simulink model "c2837xD_lcd_display"  (R2021b)
settings: Solver=FixedStepDiscrete  StartTime=0.0  StopTime=Inf  RelTol=1e-3  EnableMultiTasking=on
InitFcn:
  | c2837xD_Display_Param;
values from neighbouring files (symbols this model uses):
  SCI_counter = SCI_ping_buffer_size/SCI_chunk_size    (= 640)    [c2837xD_Display_Param.m]
  SCI_ping_buffer_size = image_height*lines_in_packet    (= 3840)    [c2837xD_Display_Param.m]
  TI_chunk_size = SCI_chunk_size    (= 6)    [c2837xD_Display_Param.m]
  TI_ping_buffer_size = SCI_ping_buffer_size    (= 3840)    [c2837xD_Display_Param.m]
libraries: c280xlib x63, c2837xDlib x63, simulink x41, c2000lib x1, demo_controls x1, dspswit3 x1, idelinklib_common x1
(part 1 of 4)
CloseFcn:
  | clearvars Image_Array image_height image_width lines_in_packet;
  | clearvars SCI_chunk_size SCI_counter SCI_ping_buffer_size;
  | clearvars SPI_chunk_size TI_chunk_size TI_ping_buffer_size;
  | clearvars ACK_array ACK_watchdog delimiter;
  | clearvars I IB IG Image inc1 inc2 IR IRG IRGB serial_obj CurrentBufferData CurrentBuffercount;
settings Model: ExtModeTrigDuration=8  Creator=The MathWorks, Inc.  LastModifiedBy=The MathWorks, Inc.
settings SolverCC: AlgebraicLoopSolver=TrustRegion
settings DataIOCC: ReturnWorkspaceOutputs=off
settings OptimizationCC: DefaultUnderspecifiedDataType=single  PassReuseOutputArgsAs=Individual arguments  MaxStackSize=512  EfficientTunableParamExpr=on
settings DebuggingCC: InheritedTsInSrcMsg=none  ParameterTunabilityLossMsg=error  SFMachineParentedDataDiag=warning  ArithmeticOperatorsInVariantConditions=warning
settings HardwareCC: ProdBitPerChar=16  ProdBitPerInt=16  ProdBitPerPointer=32  ProdBitPerSizeT=32  ProdBitPerPtrDiffT=32  ProdLargestAtomicInteger=Integer  ProdLargestAtomicFloat=None  ProdWordSize=16  ProdLongLongMode=on  ProdHWDeviceType=Texas Instruments->C2000
settings SFSimCC: SimUseLocalCustomCode=off  MATLABDynamicMemAlloc=off  CustomCodeUndefinedFunction=UseInterfaceOnly
settings RTWCC: Description=Embedded Coder  SystemTargetFile=ert.tlc  HardwareBoard=TI Delfino F28379D LaunchPad  TemplateMakefile=ert_default_tmf  GenerateReport=on  RTWUseLocalCustomCode=off  Toolchain=Texas Instruments Code Composer Studio (C2000)  IncludeHyperlinkInReport=on  LaunchReport=on  GenerateTraceInfo=on  GenerateTraceReport=on  GenerateTraceReportSl=on  GenerateTraceReportSf=on  GenerateTraceReportEml=on
settings CodeAppCC: ForceParamTrailComments=on  IgnoreCustomStorageClasses=off  OperatorAnnotations=on  SimulinkDataObjDesc=on  SFDataObjDesc=on  InsertBlockDesc=on
settings ERTTargetCC: CodeReplacementLibrary=TI C28x  MemSecPackage=tic2000demospkg  MemSecFuncExecute=code_ramfuncs

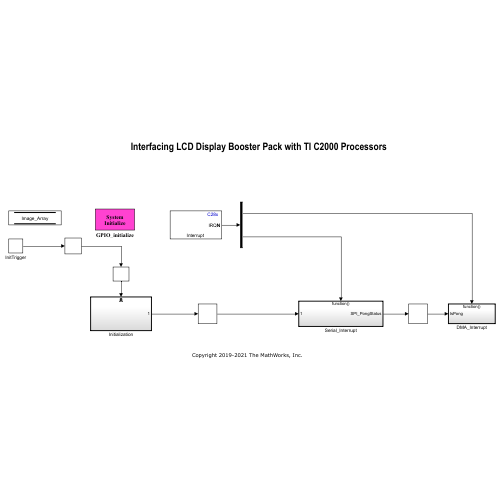
[thumbnail: Simulink's stored preview of the top-level diagram]
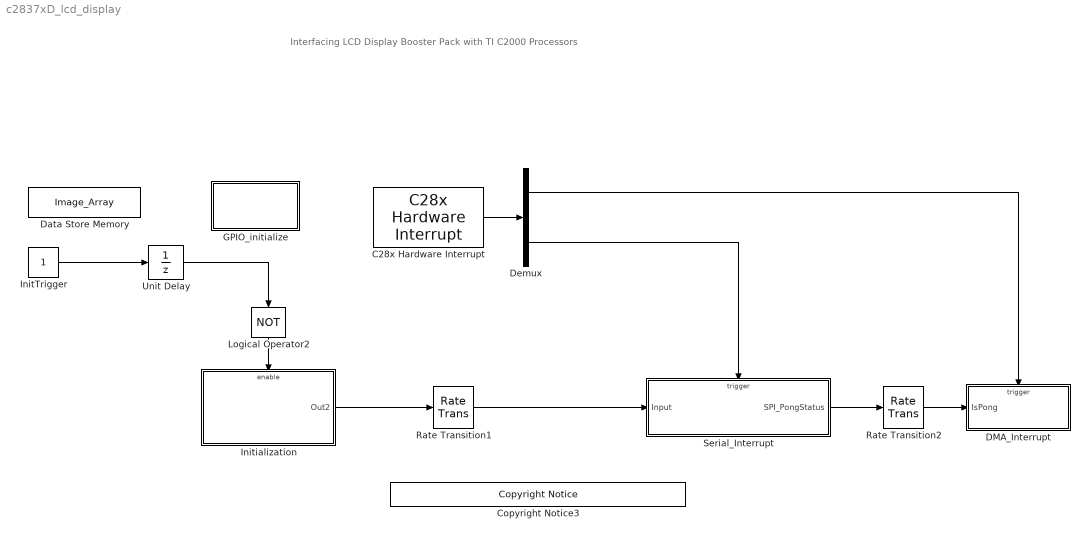
== system c2837xD_lcd_display ==
  note: Interfacing LCD Display Booster Pack with TI C2000 Processors
  C28x Hardware Interrupt : c2000lib/Scheduling/C28x Hardware Interrupt  irqnumbers=[7 9]  pienumbers=[1 1]  irqpriorities=[30 31]  irqpreempts=[1 0]  showinput=off  dspchiptype=C280X
      settings: SourceProductBaseCode=TIC2000
  Copyright Notice3 : demo_controls/Copyright Notice  year=2019  prod=tic2000
      settings: SourceProductBaseCode=ME
  DMA_Interrupt : Subsystem  TreatAsAtomicUnit=on
  Data Store Memory : DataStoreMemory  DataStoreName=Image_Array  ReadBeforeWriteMsg=warning  WriteAfterWriteMsg=warning  WriteAfterReadMsg=warning  InitialValue=[]  ShowAdditionalParam=off  OutDataTypeStr=uint16  Dimensions=SCI_ping_buffer_size*2  StateMustResolveToSignalObject=on
  Demux : Demux  Outputs=2
  GPIO_initialize : Subsystem  mask(System Initialize){ShowInLibBrowser=0}
      mask prompts: ShowInLibBrowser "Simulink:masks:CustCodeMaskParam1_MP"
      settings: CopyFcn=cccopyfcn(gcb)  OpenFcn=ccopenfcn('System Initialize Function')
      mask Help: eval('feval(''rtwprivate'',''rtwhelpview'',''rtw_sys_initialize_block'')');
      mask Display: disp('System\nInitialize');
  InitTrigger : Constant  OutDataTypeStr=uint16  SampleTime=0.1
  Initialization : Subsystem
  Logical Operator2 : Logic  Priority=2  Operator=NOT  AllPortsSameDT=off  OutDataTypeStr=boolean
  Rate Transition1 : RateTransition  Integrity=off
  Rate Transition2 : RateTransition  Integrity=off
  Serial_Interrupt : Subsystem  TreatAsAtomicUnit=on
      settings: RTWSystemCode=Nonreusable function
  Unit Delay : UnitDelay  Priority=1  SampleTime=-1  HasFrameUpgradeWarning=on
  wires:
  Initialization/1(Out2) -> Rate Transition1/1
  Demux/1 -> DMA_Interrupt/Trigger
  Demux/2 -> Serial_Interrupt/Trigger
  Logical Operator2/1 -> Initialization/Enable
  Unit Delay/1 -> Logical Operator2/1
  Rate Transition1/1 -> Serial_Interrupt/1(Input)
  InitTrigger/1 -> Unit Delay/1
  C28x Hardware Interrupt/1 -> Demux/1
  Serial_Interrupt/1(SPI_PongStatus) -> Rate Transition2/1
  Rate Transition2/1 -> DMA_Interrupt/1(IsPong)

== system c2837xD_lcd_display/DMA_Interrupt ==
  IsPong : Inport
  function : TriggerPort  TriggerType=function-call  VariantControl=Variant
  ACKCounter : simulink/Sources/Counter Free-Running  NumBits=16  tsamp=-1
  NOT : Logic  Operator=NOT  IconShape=distinctive  AllPortsSameDT=off  OutDataTypeStr=boolean
  SCI Transmit : c280xlib/SCI Transmit  sciModule=A  dataHead='S'  dataTail='E'  postInterrupt=off  numFifo=1
  Subsystem : Subsystem
  Subsystem1 : Subsystem
  wires:
  ACKCounter/1 -> SCI Transmit/1
  IsPong/1 -> Subsystem1/Enable, NOT/1
  NOT/1 -> Subsystem/Enable

== system c2837xD_lcd_display/GPIO_initialize ==

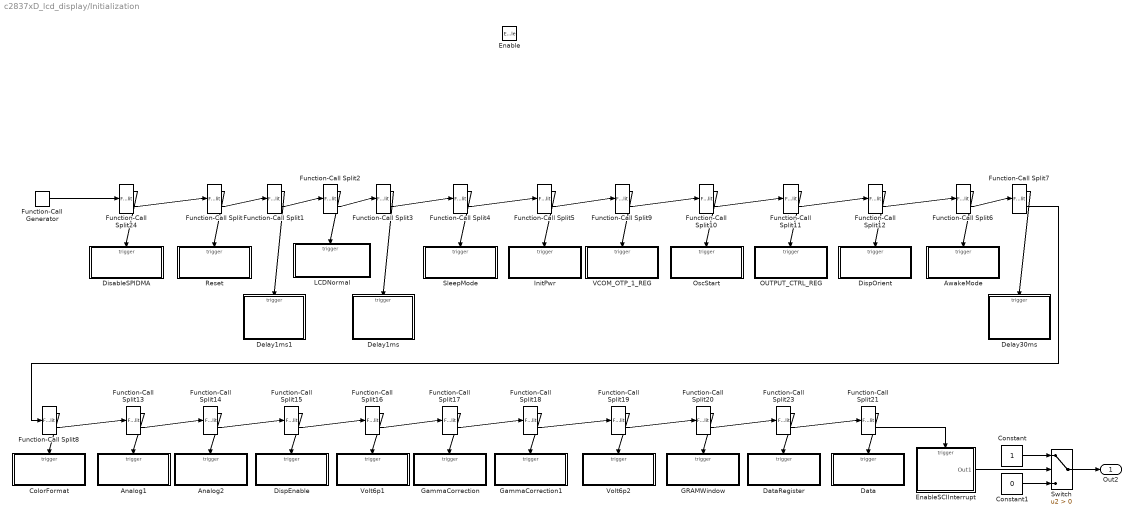
== system c2837xD_lcd_display/Initialization ==
  Enable : EnablePort
  Analog1 : Subsystem  TreatAsAtomicUnit=on
  Analog2 : Subsystem  TreatAsAtomicUnit=on
  AwakeMode : Subsystem  TreatAsAtomicUnit=on
  ColorFormat : Subsystem  TreatAsAtomicUnit=on
  Constant : Constant
  Constant1 : Constant  Value=0
  Data : Subsystem  TreatAsAtomicUnit=on
  DataRegister : Subsystem  TreatAsAtomicUnit=on
  Delay1ms : Subsystem  TreatAsAtomicUnit=on
  Delay1ms1 : Subsystem  TreatAsAtomicUnit=on
  Delay30ms : Subsystem  TreatAsAtomicUnit=on
  DisableSPIDMA : Subsystem  TreatAsAtomicUnit=on
  DispEnable : Subsystem  TreatAsAtomicUnit=on
  DispOrient : Subsystem  TreatAsAtomicUnit=on
  EnableSCIInterrupt : Subsystem  TreatAsAtomicUnit=on
  Function-Call Generator : simulink/Ports & Subsystems/Function-Call Generator  sample_time=-1  numberOfIterations=1  DisallowWideOutput=off
  Function-Call Split{,1..21,23..24} (24 alike) : FunctionCallSplit  NumOutputPorts=2
  GRAMWindow : Subsystem  TreatAsAtomicUnit=on
  GammaCorrection : Subsystem  TreatAsAtomicUnit=on
  GammaCorrection1 : Subsystem  TreatAsAtomicUnit=on
  InitPwr : Subsystem  TreatAsAtomicUnit=on
  LCDNormal : Subsystem
  OUTPUT_CTRL_REG : Subsystem  TreatAsAtomicUnit=on
  OscStart : Subsystem  TreatAsAtomicUnit=on
  Reset : Subsystem  TreatAsAtomicUnit=on
  SleepMode : Subsystem  TreatAsAtomicUnit=on
  Switch : Switch  Criteria=u2 > Threshold
  VCOM_OTP_1_REG : Subsystem  TreatAsAtomicUnit=on
  Volt6p1 : Subsystem  TreatAsAtomicUnit=on
  Volt6p2 : Subsystem  TreatAsAtomicUnit=on
  Out2 : Outport  VectorParamsAs1DForOutWhenUnconnected=off
  wires:
  Function-Call Split6/2 -> Function-Call Split7/1
  Function-Call Split19/1 -> Volt6p2/Trigger
  Function-Call Split24/1 -> DisableSPIDMA/Trigger
  Function-Call Split10/2 -> Function-Call Split11/1
  Function-Call Split10/1 -> OscStart/Trigger
  Function-Call Split21/2 -> EnableSCIInterrupt/Trigger
  Function-Call Split9/1 -> VCOM_OTP_1_REG/Trigger
  Function-Call Split1/1 -> Delay1ms1/Trigger
  Function-Call Split17/2 -> Function-Call Split18/1
  Function-Call Generator/1 -> Function-Call Split24/1
  Function-Call Split15/1 -> DispEnable/Trigger
  Function-Call Split/2 -> Function-Call Split1/1
  Function-Call Split12/1 -> DispOrient/Trigger
  Function-Call Split5/2 -> Function-Call Split9/1
  EnableSCIInterrupt/1(Out1) -> Switch/2
  Function-Call Split7/1 -> Delay30ms/Trigger
  Function-Call Split23/2 -> Function-Call Split21/1
  Function-Call Split2/1 -> LCDNormal/Trigger
  Function-Call Split2/2 -> Function-Call Split3/1
  Function-Call Split5/1 -> InitPwr/Trigger
  Constant1/1 -> Switch/3
  Function-Call Split11/1 -> OUTPUT_CTRL_REG/Trigger
  Function-Call Split21/1 -> Data/Trigger
  Function-Call Split1/2 -> Function-Call Split2/1
  Function-Call Split8/1 -> ColorFormat/Trigger
  Function-Call Split17/1 -> GammaCorrection/Trigger
  Function-Call Split16/2 -> Function-Call Split17/1
  Function-Call Split18/2 -> Function-Call Split19/1
  Function-Call Split/1 -> Reset/Trigger
  Function-Call Split13/2 -> Function-Call Split14/1
  Function-Call Split11/2 -> Function-Call Split12/1
  Function-Call Split14/2 -> Function-Call Split15/1
  Function-Call Split16/1 -> Volt6p1/Trigger
  Function-Call Split8/2 -> Function-Call Split13/1
  Function-Call Split7/2 -> Function-Call Split8/1
  Function-Call Split13/1 -> Analog1/Trigger
  Function-Call Split6/1 -> AwakeMode/Trigger
  Function-Call Split18/1 -> GammaCorrection1/Trigger
  Function-Call Split14/1 -> Analog2/Trigger
  Function-Call Split20/2 -> Function-Call Split23/1
  Function-Call Split20/1 -> GRAMWindow/Trigger
  Function-Call Split24/2 -> Function-Call Split/1
  Function-Call Split19/2 -> Function-Call Split20/1
  Function-Call Split15/2 -> Function-Call Split16/1
  Function-Call Split4/1 -> SleepMode/Trigger
  Function-Call Split3/1 -> Delay1ms/Trigger
  Constant/1 -> Switch/1
  Switch/1 -> Out2/1
  Function-Call Split4/2 -> Function-Call Split5/1
  Function-Call Split3/2 -> Function-Call Split4/1
  Function-Call Split12/2 -> Function-Call Split6/1
  Function-Call Split23/1 -> DataRegister/Trigger
  Function-Call Split9/2 -> Function-Call Split10/1

== system c2837xD_lcd_display/Serial_Interrupt ==
  Input : Inport
  function : TriggerPort  TriggerType=function-call  VariantControl=Variant
  SCIInterruptEnable : Subsystem
  SPI_PongStatus : Outport  VectorParamsAs1DForOutWhenUnconnected=off
  wires:
  SCIInterruptEnable/1(SPI_PongStatus) -> SPI_PongStatus/1
  Input/1 -> SCIInterruptEnable/Enable

== system c2837xD_lcd_display/DMA_Interrupt/Subsystem ==
  Enable : EnablePort
  changeAddress : Subsystem  mask(System Outputs){ShowInLibBrowser=0}
      mask prompts: ShowInLibBrowser "Simulink:masks:CustCodeMaskParam1_MP"
      settings: CopyFcn=cccopyfcn(gcb)  OpenFcn=ccopenfcn('System Outputs Function')
      mask Help: eval('feval(''rtwprivate'',''rtwhelpview'',''rtw_sys_outputs_block'')');
      mask Display: disp('System\nOutputs');

== system c2837xD_lcd_display/DMA_Interrupt/Subsystem1 ==
  Enable : EnablePort
  changeAddress : Subsystem  mask(System Outputs){ShowInLibBrowser=0}
      mask prompts: ShowInLibBrowser "Simulink:masks:CustCodeMaskParam1_MP"
      settings: CopyFcn=cccopyfcn(gcb)  OpenFcn=ccopenfcn('System Outputs Function')
      mask Help: eval('feval(''rtwprivate'',''rtwhelpview'',''rtw_sys_outputs_block'')');
      mask Display: disp('System\nOutputs');

== system c2837xD_lcd_display/Initialization/Analog1 ==
  function : TriggerPort  TriggerType=function-call  VariantControl=Variant
  Constant2 : Constant  Value=hex2dec('12')  OutDataTypeStr=uint16  SampleTime=-1
  Constant3 : Constant  Value=[hex2dec('09') hex2dec('99')]  OutDataTypeStr=uint16  SampleTime=-1
  Subsystem : Subsystem
  wires:
  Constant3/1 -> Subsystem/2(Data)
  Constant2/1 -> Subsystem/1(Cmd)

== system c2837xD_lcd_display/Initialization/Analog2 ==
  function : TriggerPort  TriggerType=function-call  VariantControl=Variant
  Constant2 : Constant  Value=hex2dec('26')  OutDataTypeStr=uint16  SampleTime=-1
  Constant3 : Constant  Value=[hex2dec('38') hex2dec('00')]  OutDataTypeStr=uint16  SampleTime=-1
  Subsystem : Subsystem
  wires:
  Constant3/1 -> Subsystem/2(Data)
  Constant2/1 -> Subsystem/1(Cmd)

== system c2837xD_lcd_display/Initialization/AwakeMode ==
  function : TriggerPort  TriggerType=function-call  VariantControl=Variant
  Constant2 : Constant  Value=hex2dec('10')  OutDataTypeStr=uint16  SampleTime=-1
  Constant3 : Constant  Value=[hex2dec('00') hex2dec('00')]  OutDataTypeStr=uint16  SampleTime=-1
  Subsystem : Subsystem
  wires:
  Constant2/1 -> Subsystem/1(Cmd)
  Constant3/1 -> Subsystem/2(Data)

== system c2837xD_lcd_display/Initialization/ColorFormat ==
  function : TriggerPort  TriggerType=function-call  VariantControl=Variant
  Constant2 : Constant  Value=hex2dec('11')  OutDataTypeStr=uint16  SampleTime=-1
  Constant5 : Constant  Value=[hex2dec('62') hex2dec('38')]  OutDataTypeStr=uint16  SampleTime=-1
  Subsystem : Subsystem
  wires:
  Constant2/1 -> Subsystem/1(Cmd)
  Constant5/1 -> Subsystem/2(Data)

== system c2837xD_lcd_display/Initialization/Data ==
  function : TriggerPort  TriggerType=function-call  VariantControl=Variant
  Constant : Constant  Value=hex2dec('22')  OutDataTypeStr=uint16  SampleTime=-1
  LCD Data : Subsystem  TreatAsAtomicUnit=on  RTWFcnName=writeLCDData  RTWFileName=write_data
      settings: RTWFcnNameOpts=User specified
  wires:
  Constant/1 -> LCD Data/1(Cmd)

== system c2837xD_lcd_display/Initialization/DataRegister ==
  function : TriggerPort  TriggerType=function-call  VariantControl=Variant
  Constant : Constant  Value=hex2dec('22')  OutDataTypeStr=uint16  SampleTime=-1
  Constant4 : Constant  Value=[hex2dec('07') hex2dec('E0')]  OutDataTypeStr=uint16  SampleTime=-1
  LCD Data : Subsystem  TreatAsAtomicUnit=on  RTWFcnName=writeLCDData  RTWFileName=write_data
      settings: RTWFcnNameOpts=User specified
  wires:
  Constant/1 -> LCD Data/1(Cmd)
  Constant4/1 -> LCD Data/2(Data)

== system c2837xD_lcd_display/Initialization/Delay1ms ==
  function : TriggerPort  TriggerType=function-call  VariantControl=Variant
  System Outputs : Subsystem  mask(System Outputs){ShowInLibBrowser=0}
      mask prompts: ShowInLibBrowser "Simulink:masks:CustCodeMaskParam1_MP"
      settings: CopyFcn=cccopyfcn(gcb)  OpenFcn=ccopenfcn('System Outputs Function')
      mask Help: eval('feval(''rtwprivate'',''rtwhelpview'',''rtw_sys_outputs_block'')');
      mask Display: disp('System\nOutputs');

== system c2837xD_lcd_display/Initialization/Delay1ms1 ==
  function : TriggerPort  TriggerType=function-call  VariantControl=Variant
  System Outputs : Subsystem  mask(System Outputs){ShowInLibBrowser=0}
      mask prompts: ShowInLibBrowser "Simulink:masks:CustCodeMaskParam1_MP"
      settings: CopyFcn=cccopyfcn(gcb)  OpenFcn=ccopenfcn('System Outputs Function')
      mask Help: eval('feval(''rtwprivate'',''rtwhelpview'',''rtw_sys_outputs_block'')');
      mask Display: disp('System\nOutputs');

== system c2837xD_lcd_display/Initialization/Delay30ms ==
  function : TriggerPort  TriggerType=function-call  VariantControl=Variant
  System Outputs : Subsystem  mask(System Outputs){ShowInLibBrowser=0}
      mask prompts: ShowInLibBrowser "Simulink:masks:CustCodeMaskParam1_MP"
      settings: CopyFcn=cccopyfcn(gcb)  OpenFcn=ccopenfcn('System Outputs Function')
      mask Help: eval('feval(''rtwprivate'',''rtwhelpview'',''rtw_sys_outputs_block'')');
      mask Display: disp('System\nOutputs');

== system c2837xD_lcd_display/Initialization/DisableSPIDMA ==
  function : TriggerPort  TriggerType=function-call  VariantControl=Variant
  Disable SPIDMAA : Subsystem  mask(System Outputs){ShowInLibBrowser=0}
      mask prompts: ShowInLibBrowser "Simulink:masks:CustCodeMaskParam1_MP"
      settings: CopyFcn=cccopyfcn(gcb)  OpenFcn=ccopenfcn('System Outputs Function')
      mask Help: eval('feval(''rtwprivate'',''rtwhelpview'',''rtw_sys_outputs_block'')');
      mask Display: disp('System\nOutputs');

== system c2837xD_lcd_display/Initialization/DispEnable ==
  function : TriggerPort  TriggerType=function-call  VariantControl=Variant
  Constant2 : Constant  Value=hex2dec('07')  OutDataTypeStr=uint16  SampleTime=-1
  Constant3 : Constant  Value=[hex2dec('00') hex2dec('33')]  OutDataTypeStr=uint16  SampleTime=-1
  Subsystem : Subsystem
  wires:
  Constant2/1 -> Subsystem/1(Cmd)
  Constant3/1 -> Subsystem/2(Data)

== system c2837xD_lcd_display/Initialization/DispOrient ==
  function : TriggerPort  TriggerType=function-call  VariantControl=Variant
  Constant2 : Constant  Value=hex2dec('02')  OutDataTypeStr=uint16  SampleTime=-1
  Constant3 : Constant  Value=[hex2dec('06') hex2dec('00')]  OutDataTypeStr=uint16  SampleTime=-1
  Subsystem : Subsystem
  wires:
  Constant3/1 -> Subsystem/2(Data)
  Constant2/1 -> Subsystem/1(Cmd)

== system c2837xD_lcd_display/Initialization/EnableSCIInterrupt ==
  function : TriggerPort  TriggerType=function-call  VariantControl=Variant
  Constant : Constant
  SPISettings : Subsystem  mask(System Outputs){ShowInLibBrowser=0}
      mask prompts: ShowInLibBrowser "Simulink:masks:CustCodeMaskParam1_MP"
      settings: CopyFcn=cccopyfcn(gcb)  OpenFcn=ccopenfcn('System Outputs Function')
      mask Help: eval('feval(''rtwprivate'',''rtwhelpview'',''rtw_sys_outputs_block'')');
      mask Display: disp('System\nOutputs');
  Out1 : Outport  VectorParamsAs1DForOutWhenUnconnected=off
  wires:
  Constant/1 -> Out1/1

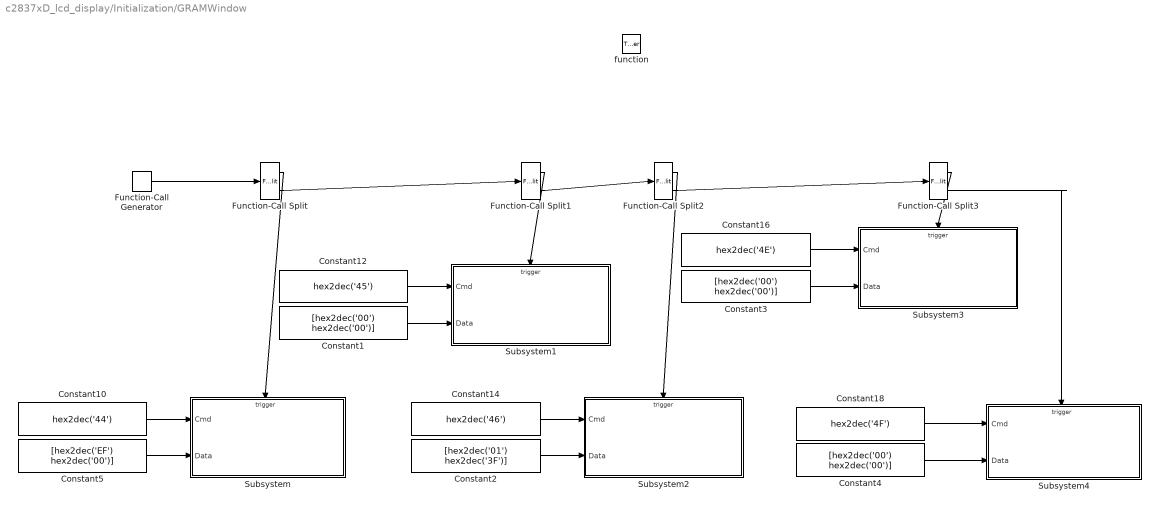
== system c2837xD_lcd_display/Initialization/GRAMWindow ==
  function : TriggerPort  TriggerType=function-call  VariantControl=Variant
  Constant1 : Constant  Value=[hex2dec('00') hex2dec('00')]  OutDataTypeStr=uint16  SampleTime=-1
  Constant10 : Constant  Value=hex2dec('44')  OutDataTypeStr=uint16  SampleTime=-1
  Constant12 : Constant  Value=hex2dec('45')  OutDataTypeStr=uint16  SampleTime=-1
  Constant14 : Constant  Value=hex2dec('46')  OutDataTypeStr=uint16  SampleTime=-1
  Constant16 : Constant  Value=hex2dec('4E')  OutDataTypeStr=uint16  SampleTime=-1
  Constant18 : Constant  Value=hex2dec('4F')  OutDataTypeStr=uint16  SampleTime=-1
  Constant2 : Constant  Value=[hex2dec('01') hex2dec('3F')]  OutDataTypeStr=uint16  SampleTime=-1
  Constant3 : Constant  Value=[hex2dec('00') hex2dec('00')]  OutDataTypeStr=uint16  SampleTime=-1
  Constant4 : Constant  Value=[hex2dec('00') hex2dec('00')]  OutDataTypeStr=uint16  SampleTime=-1
  Constant5 : Constant  Value=[hex2dec('EF') hex2dec('00')]  OutDataTypeStr=uint16  SampleTime=-1
  Function-Call Generator : simulink/Ports & Subsystems/Function-Call Generator  sample_time=-1  numberOfIterations=1  DisallowWideOutput=off
  Function-Call Split{,1..3} (4 alike) : FunctionCallSplit  NumOutputPorts=2
  Subsystem : Subsystem
  Subsystem1 : Subsystem
  Subsystem2 : Subsystem
  Subsystem3 : Subsystem
  Subsystem4 : Subsystem
  wires:
  Function-Call Split/1 -> Subsystem/Trigger
  Function-Call Generator/1 -> Function-Call Split/1
  Function-Call Split/2 -> Function-Call Split1/1
  Function-Call Split1/2 -> Function-Call Split2/1
  Function-Call Split1/1 -> Subsystem1/Trigger
  Function-Call Split2/2 -> Function-Call Split3/1
  Function-Call Split2/1 -> Subsystem2/Trigger
  Function-Call Split3/2 -> Subsystem4/Trigger
  Function-Call Split3/1 -> Subsystem3/Trigger
  Constant5/1 -> Subsystem/2(Data)
  Constant10/1 -> Subsystem/1(Cmd)
  Constant1/1 -> Subsystem1/2(Data)
  Constant12/1 -> Subsystem1/1(Cmd)
  Constant2/1 -> Subsystem2/2(Data)
  Constant14/1 -> Subsystem2/1(Cmd)
  Constant3/1 -> Subsystem3/2(Data)
  Constant16/1 -> Subsystem3/1(Cmd)
  Constant18/1 -> Subsystem4/1(Cmd)
  Constant4/1 -> Subsystem4/2(Data)

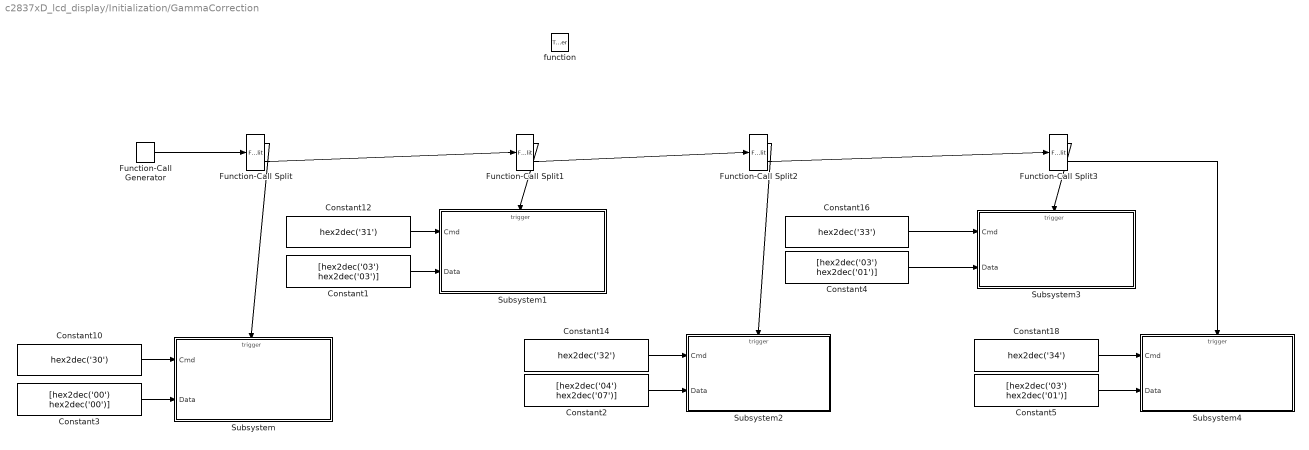
== system c2837xD_lcd_display/Initialization/GammaCorrection ==
  function : TriggerPort  TriggerType=function-call  VariantControl=Variant
  Constant1 : Constant  Value=[hex2dec('03') hex2dec('03')]  OutDataTypeStr=uint16  SampleTime=-1
  Constant10 : Constant  Value=hex2dec('30')  OutDataTypeStr=uint16  SampleTime=-1
  Constant12 : Constant  Value=hex2dec('31')  OutDataTypeStr=uint16  SampleTime=-1
  Constant14 : Constant  Value=hex2dec('32')  OutDataTypeStr=uint16  SampleTime=-1
  Constant16 : Constant  Value=hex2dec('33')  OutDataTypeStr=uint16  SampleTime=-1
  Constant18 : Constant  Value=hex2dec('34')  OutDataTypeStr=uint16  SampleTime=-1
  Constant2 : Constant  Value=[hex2dec('04') hex2dec('07')]  OutDataTypeStr=uint16  SampleTime=-1
  Constant3 : Constant  Value=[hex2dec('00') hex2dec('00')]  OutDataTypeStr=uint16  SampleTime=-1
  Constant4 : Constant  Value=[hex2dec('03') hex2dec('01')]  OutDataTypeStr=uint16  SampleTime=-1
  Constant5 : Constant  Value=[hex2dec('03') hex2dec('01')]  OutDataTypeStr=uint16  SampleTime=-1
  Function-Call Generator : simulink/Ports & Subsystems/Function-Call Generator  sample_time=-1  numberOfIterations=1  DisallowWideOutput=off
  Function-Call Split{,1..3} (4 alike) : FunctionCallSplit  NumOutputPorts=2
  Subsystem : Subsystem
  Subsystem1 : Subsystem
  Subsystem2 : Subsystem
  Subsystem3 : Subsystem
  Subsystem4 : Subsystem
  wires:
  Function-Call Generator/1 -> Function-Call Split/1
  Function-Call Split/1 -> Subsystem/Trigger
  Function-Call Split/2 -> Function-Call Split1/1
  Function-Call Split1/1 -> Subsystem1/Trigger
  Function-Call Split1/2 -> Function-Call Split2/1
  Function-Call Split2/1 -> Subsystem2/Trigger
  Function-Call Split2/2 -> Function-Call Split3/1
  Function-Call Split3/1 -> Subsystem3/Trigger
  Function-Call Split3/2 -> Subsystem4/Trigger
  Constant3/1 -> Subsystem/2(Data)
  Constant10/1 -> Subsystem/1(Cmd)
  Constant1/1 -> Subsystem1/2(Data)
  Constant12/1 -> Subsystem1/1(Cmd)
  Constant2/1 -> Subsystem2/2(Data)
  Constant14/1 -> Subsystem2/1(Cmd)
  Constant4/1 -> Subsystem3/2(Data)
  Constant16/1 -> Subsystem3/1(Cmd)
  Constant5/1 -> Subsystem4/2(Data)
  Constant18/1 -> Subsystem4/1(Cmd)

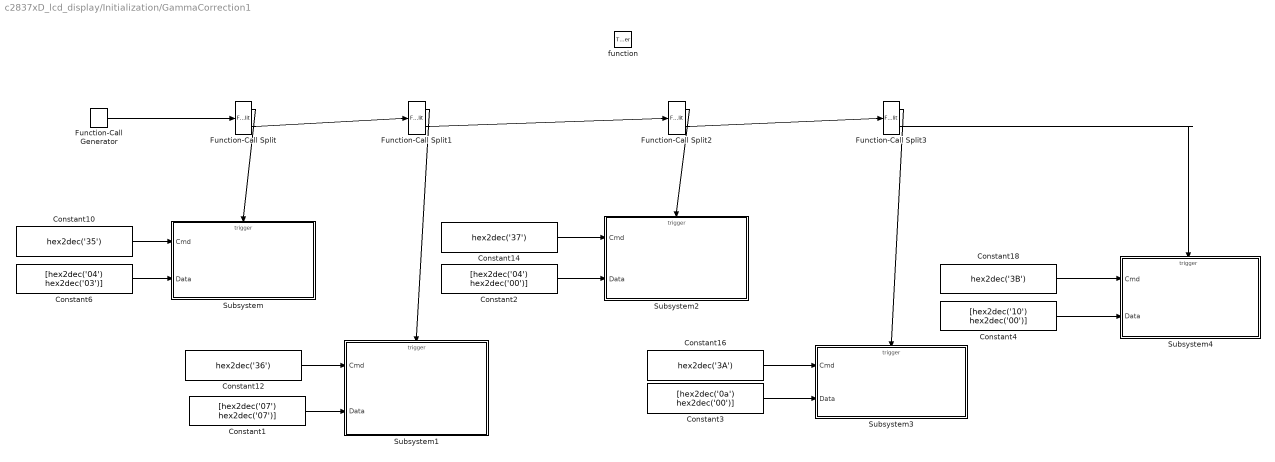
== system c2837xD_lcd_display/Initialization/GammaCorrection1 ==
  function : TriggerPort  TriggerType=function-call  VariantControl=Variant
  Constant1 : Constant  Value=[hex2dec('07') hex2dec('07')]  OutDataTypeStr=uint16  SampleTime=-1
  Constant10 : Constant  Value=hex2dec('35')  OutDataTypeStr=uint16  SampleTime=-1
  Constant12 : Constant  Value=hex2dec('36')  OutDataTypeStr=uint16  SampleTime=-1
  Constant14 : Constant  Value=hex2dec('37')  OutDataTypeStr=uint16  SampleTime=-1
  Constant16 : Constant  Value=hex2dec('3A')  OutDataTypeStr=uint16  SampleTime=-1
  Constant18 : Constant  Value=hex2dec('3B')  OutDataTypeStr=uint16  SampleTime=-1
  Constant2 : Constant  Value=[hex2dec('04') hex2dec('00')]  OutDataTypeStr=uint16  SampleTime=-1
  Constant3 : Constant  Value=[hex2dec('0a') hex2dec('00')]  OutDataTypeStr=uint16  SampleTime=-1
  Constant4 : Constant  Value=[hex2dec('10') hex2dec('00')]  OutDataTypeStr=uint16  SampleTime=-1
  Constant6 : Constant  Value=[hex2dec('04') hex2dec('03')]  OutDataTypeStr=uint16  SampleTime=-1
  Function-Call Generator : simulink/Ports & Subsystems/Function-Call Generator  sample_time=-1  numberOfIterations=1  DisallowWideOutput=off
  Function-Call Split{,1..3} (4 alike) : FunctionCallSplit  NumOutputPorts=2
  Subsystem : Subsystem
  Subsystem1 : Subsystem
  Subsystem2 : Subsystem
  Subsystem3 : Subsystem
  Subsystem4 : Subsystem
  wires:
  Function-Call Generator/1 -> Function-Call Split/1
  Function-Call Split/1 -> Subsystem/Trigger
  Function-Call Split/2 -> Function-Call Split1/1
  Function-Call Split1/2 -> Function-Call Split2/1
  Function-Call Split2/2 -> Function-Call Split3/1
  Function-Call Split3/2 -> Subsystem4/Trigger
  Function-Call Split3/1 -> Subsystem3/Trigger
  Function-Call Split1/1 -> Subsystem1/Trigger
  Function-Call Split2/1 -> Subsystem2/Trigger
  Constant6/1 -> Subsystem/2(Data)
  Constant10/1 -> Subsystem/1(Cmd)
  Constant12/1 -> Subsystem1/1(Cmd)
  Constant1/1 -> Subsystem1/2(Data)
  Constant2/1 -> Subsystem2/2(Data)
  Constant14/1 -> Subsystem2/1(Cmd)
  Constant16/1 -> Subsystem3/1(Cmd)
  Constant3/1 -> Subsystem3/2(Data)
  Constant4/1 -> Subsystem4/2(Data)
  Constant18/1 -> Subsystem4/1(Cmd)

== system c2837xD_lcd_display/Initialization/InitPwr ==
  function : TriggerPort  TriggerType=function-call  VariantControl=Variant
  Constant2 : Constant  Value=hex2dec('1E')  OutDataTypeStr=uint16  SampleTime=-1
  Constant5 : Constant  Value=[hex2dec('00') hex2dec('B2')]  OutDataTypeStr=uint16  SampleTime=-1
  Subsystem : Subsystem
  wires:
  Constant2/1 -> Subsystem/1(Cmd)
  Constant5/1 -> Subsystem/2(Data)

== system c2837xD_lcd_display/Initialization/LCDNormal ==
  function : TriggerPort  TriggerType=function-call  VariantControl=Variant
  System Outputs1 : Subsystem  mask(System Outputs){ShowInLibBrowser=0}
      mask prompts: ShowInLibBrowser "Simulink:masks:CustCodeMaskParam1_MP"
      settings: CopyFcn=cccopyfcn(gcb)  OpenFcn=ccopenfcn('System Outputs Function')
      mask Help: eval('feval(''rtwprivate'',''rtwhelpview'',''rtw_sys_outputs_block'')');
      mask Display: disp('System\nOutputs');

== system c2837xD_lcd_display/Initialization/OUTPUT_CTRL_REG ==
  function : TriggerPort  TriggerType=function-call  VariantControl=Variant
  Constant2 : Constant  Value=hex2dec('01')  OutDataTypeStr=uint16  SampleTime=-1
  Constant3 : Constant  Value=[hex2dec('30') hex2dec('EF')]  OutDataTypeStr=uint16  SampleTime=-1
  Subsystem : Subsystem
  wires:
  Constant3/1 -> Subsystem/2(Data)
  Constant2/1 -> Subsystem/1(Cmd)

== system c2837xD_lcd_display/Initialization/OscStart ==
  function : TriggerPort  TriggerType=function-call  VariantControl=Variant
  Constant2 : Constant  Value=hex2dec('00')  OutDataTypeStr=uint16  SampleTime=-1
  Constant3 : Constant  Value=[hex2dec('00') hex2dec('01')]  OutDataTypeStr=uint16  SampleTime=-1
  Subsystem : Subsystem
  wires:
  Constant3/1 -> Subsystem/2(Data)
  Constant2/1 -> Subsystem/1(Cmd)

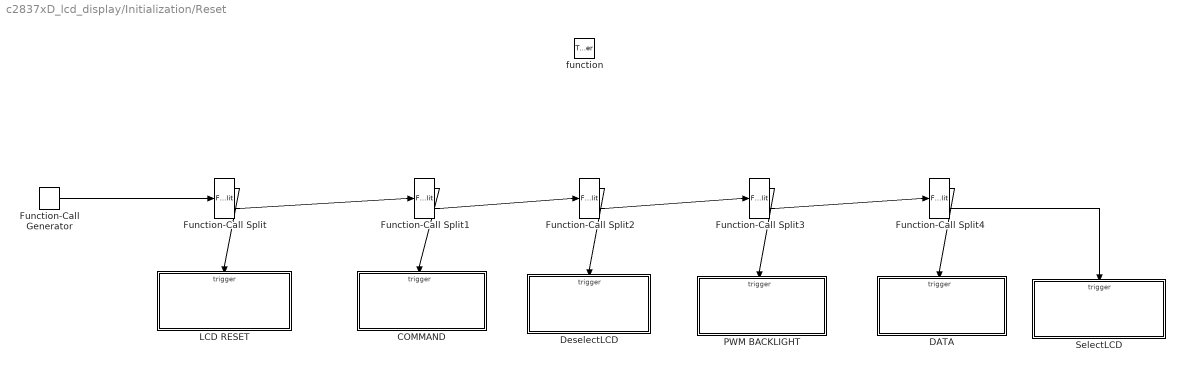
== system c2837xD_lcd_display/Initialization/Reset ==
  function : TriggerPort  TriggerType=function-call  VariantControl=Variant
  COMMAND : Subsystem
  DATA : Subsystem
  DeselectLCD : Subsystem
  Function-Call Generator : simulink/Ports & Subsystems/Function-Call Generator  sample_time=-1  numberOfIterations=1  DisallowWideOutput=off
  Function-Call Split{,1..4} (5 alike) : FunctionCallSplit  NumOutputPorts=2
  LCD RESET : Subsystem
  PWM BACKLIGHT : Subsystem
  SelectLCD : Subsystem
  wires:
  Function-Call Generator/1 -> Function-Call Split/1
  Function-Call Split/1 -> LCD RESET/Trigger
  Function-Call Split/2 -> Function-Call Split1/1
  Function-Call Split1/1 -> COMMAND/Trigger
  Function-Call Split1/2 -> Function-Call Split2/1
  Function-Call Split2/1 -> DeselectLCD/Trigger
  Function-Call Split2/2 -> Function-Call Split3/1
  Function-Call Split3/1 -> PWM BACKLIGHT/Trigger
  Function-Call Split3/2 -> Function-Call Split4/1
  Function-Call Split4/1 -> DATA/Trigger
  Function-Call Split4/2 -> SelectLCD/Trigger

== system c2837xD_lcd_display/Initialization/SleepMode ==
  function : TriggerPort  TriggerType=function-call  VariantControl=Variant
  Data : Constant  Value=[hex2dec('00') hex2dec('01')]  OutDataTypeStr=uint16  SampleTime=-1
  SleepModeReg : Constant  Value=hex2dec('10')  OutDataTypeStr=uint16  SampleTime=-1
  Subsystem : Subsystem
  wires:
  SleepModeReg/1 -> Subsystem/1(Cmd)
  Data/1 -> Subsystem/2(Data)

== system c2837xD_lcd_display/Initialization/VCOM_OTP_1_REG ==
  function : TriggerPort  TriggerType=function-call  VariantControl=Variant
  Constant2 : Constant  Value=hex2dec('28')  OutDataTypeStr=uint16  SampleTime=-1
  Constant3 : Constant  Value=[hex2dec('00') hex2dec('06')]  OutDataTypeStr=uint16  SampleTime=-1
  Subsystem : Subsystem
  wires:
  Constant2/1 -> Subsystem/1(Cmd)
  Constant3/1 -> Subsystem/2(Data)

== system c2837xD_lcd_display/Initialization/Volt6p1 ==
  function : TriggerPort  TriggerType=function-call  VariantControl=Variant
  Constant2 : Constant  Value=hex2dec('0C')  OutDataTypeStr=uint16  SampleTime=-1
  Constant3 : Constant  Value=[hex2dec('00') hex2dec('05')]  OutDataTypeStr=uint16  SampleTime=-1
  Subsystem : Subsystem
  wires:
  Constant2/1 -> Subsystem/1(Cmd)
  Constant3/1 -> Subsystem/2(Data)

== system c2837xD_lcd_display/Initialization/Volt6p2 ==
  function : TriggerPort  TriggerType=function-call  VariantControl=Variant
  Constant1 : Constant  Value=[hex2dec('2E') hex2dec('00')]  OutDataTypeStr=uint16  SampleTime=-1
  Constant3 : Constant  Value=[hex2dec('00') hex2dec('0a')]  OutDataTypeStr=uint16  SampleTime=-1
  Constant4 : Constant  Value=hex2dec('0D')  OutDataTypeStr=uint16  SampleTime=-1
  Constant6 : Constant  Value=hex2dec('0E')  OutDataTypeStr=uint16  SampleTime=-1
  Function-Call Generator : simulink/Ports & Subsystems/Function-Call Generator  sample_time=-1  numberOfIterations=1  DisallowWideOutput=off
  Function-Call Split : FunctionCallSplit  NumOutputPorts=2
  Subsystem : Subsystem
  Subsystem1 : Subsystem
  wires:
  Function-Call Split/1 -> Subsystem/Trigger
  Function-Call Split/2 -> Subsystem1/Trigger
  Function-Call Generator/1 -> Function-Call Split/1
  Constant3/1 -> Subsystem/2(Data)
  Constant4/1 -> Subsystem/1(Cmd)
  Constant1/1 -> Subsystem1/2(Data)
  Constant6/1 -> Subsystem1/1(Cmd)

== system c2837xD_lcd_display/Serial_Interrupt/SCIInterruptEnable ==
  Enable : EnablePort
  ChangeStatus : Subsystem  Priority=20
  Counter Logic : Subsystem
  Detect Ping-Pong Change : Subsystem
  Is Matching Delimiter : Subsystem
  RecordDataIntoPingPongBuffer : Subsystem  Priority=10
  SCI Receive : c280xlib/SCI Receive  sciModule=A  dataHead=''  dataTail=''  dataType=uint16  dataDim=TI_chunk_size  initValue=0  errOption=Output the last received value  errValue=0  sampleTime=-1  outputStatus=off  postInterrupt=on  numFifo=12
      settings: SourceProductBaseCode=TIC2000
  SPI_PongStatus : Outport  VectorParamsAs1DForOutWhenUnconnected=off
  wires:
  Is Matching Delimiter/1(Out1) -> Counter Logic/1(DelimiterMatching)
  Counter Logic/3(PingPongStatus) -> ChangeStatus/1(IsPong), Detect Ping-Pong Change/1(In1), RecordDataIntoPingPongBuffer/2(IsPong)
  Counter Logic/2(CounterValue) -> RecordDataIntoPingPongBuffer/1(AddressCounter)
  Detect Ping-Pong Change/1(Out1) -> ChangeStatus/Enable
  SCI Receive/1 -> RecordDataIntoPingPongBuffer/3(Data), Is Matching Delimiter/1(In1)
  ChangeStatus/1(SPI_PongStatus) -> SPI_PongStatus/1
  Counter Logic/1(Delimiter_found) -> RecordDataIntoPingPongBuffer/Enable

== system c2837xD_lcd_display/DMA_Interrupt/Subsystem/changeAddress ==

== system c2837xD_lcd_display/DMA_Interrupt/Subsystem1/changeAddress ==

== system c2837xD_lcd_display/Initialization/Analog1/Subsystem ==
  Cmd : Inport
  Data : Inport  Port=2
  Function-Call Generator : simulink/Ports & Subsystems/Function-Call Generator  sample_time=-1  numberOfIterations=1  DisallowWideOutput=off
  Function-Call Split : FunctionCallSplit  NumOutputPorts=2
  Function-Call Split1 : FunctionCallSplit  NumOutputPorts=2
  Function-Call Split4 : FunctionCallSplit  NumOutputPorts=2
  SendCommand : Subsystem
  SendData : Subsystem
  SetCmd : Subsystem  TreatAsAtomicUnit=on
  SetData : Subsystem  TreatAsAtomicUnit=on
  wires:
  Function-Call Split1/1 -> SendCommand/Trigger
  Function-Call Generator/1 -> Function-Call Split/1
  Function-Call Split/1 -> SetCmd/Trigger
  Function-Call Split4/2 -> SendData/Trigger
  Function-Call Split4/1 -> SetData/Trigger
  Data/1 -> SendData/1(Data)
  Cmd/1 -> SendCommand/1(cmd)
  Function-Call Split1/2 -> Function-Call Split4/1
  Function-Call Split/2 -> Function-Call Split1/1

== system c2837xD_lcd_display/Initialization/Analog2/Subsystem ==
  Cmd : Inport
  Data : Inport  Port=2
  Function-Call Generator : simulink/Ports & Subsystems/Function-Call Generator  sample_time=-1  numberOfIterations=1  DisallowWideOutput=off
  Function-Call Split : FunctionCallSplit  NumOutputPorts=2
  Function-Call Split1 : FunctionCallSplit  NumOutputPorts=2
  Function-Call Split4 : FunctionCallSplit  NumOutputPorts=2
  SendCommand : Subsystem
  SendData : Subsystem
  SetCmd : Subsystem  TreatAsAtomicUnit=on
  SetData : Subsystem  TreatAsAtomicUnit=on
  wires:
  Function-Call Split1/1 -> SendCommand/Trigger
  Function-Call Generator/1 -> Function-Call Split/1
  Function-Call Split/1 -> SetCmd/Trigger
  Function-Call Split4/2 -> SendData/Trigger
  Function-Call Split4/1 -> SetData/Trigger
  Data/1 -> SendData/1(Data)
  Cmd/1 -> SendCommand/1(cmd)
  Function-Call Split1/2 -> Function-Call Split4/1
  Function-Call Split/2 -> Function-Call Split1/1

== system c2837xD_lcd_display/Initialization/AwakeMode/Subsystem ==
  Cmd : Inport
  Data : Inport  Port=2
  Function-Call Generator : simulink/Ports & Subsystems/Function-Call Generator  sample_time=-1  numberOfIterations=1  DisallowWideOutput=off
  Function-Call Split : FunctionCallSplit  NumOutputPorts=2
  Function-Call Split1 : FunctionCallSplit  NumOutputPorts=2
  Function-Call Split4 : FunctionCallSplit  NumOutputPorts=2
  SendCommand : Subsystem
  SendData : Subsystem
  SetCmd : Subsystem  TreatAsAtomicUnit=on
  SetData : Subsystem  TreatAsAtomicUnit=on
  wires:
  Function-Call Split1/1 -> SendCommand/Trigger
  Function-Call Generator/1 -> Function-Call Split/1
  Function-Call Split/1 -> SetCmd/Trigger
  Function-Call Split4/2 -> SendData/Trigger
  Function-Call Split4/1 -> SetData/Trigger
  Data/1 -> SendData/1(Data)
  Cmd/1 -> SendCommand/1(cmd)
  Function-Call Split1/2 -> Function-Call Split4/1
  Function-Call Split/2 -> Function-Call Split1/1

== system c2837xD_lcd_display/Initialization/ColorFormat/Subsystem ==
  Cmd : Inport
  Data : Inport  Port=2
  Function-Call Generator : simulink/Ports & Subsystems/Function-Call Generator  sample_time=-1  numberOfIterations=1  DisallowWideOutput=off
  Function-Call Split : FunctionCallSplit  NumOutputPorts=2
  Function-Call Split1 : FunctionCallSplit  NumOutputPorts=2
  Function-Call Split4 : FunctionCallSplit  NumOutputPorts=2
  SendCommand : Subsystem
  SendData : Subsystem
  SetCmd : Subsystem  TreatAsAtomicUnit=on
  SetData : Subsystem  TreatAsAtomicUnit=on
  wires:
  Function-Call Split1/1 -> SendCommand/Trigger
  Function-Call Generator/1 -> Function-Call Split/1
  Function-Call Split/1 -> SetCmd/Trigger
  Function-Call Split4/2 -> SendData/Trigger
  Function-Call Split4/1 -> SetData/Trigger
  Data/1 -> SendData/1(Data)
  Cmd/1 -> SendCommand/1(cmd)
  Function-Call Split1/2 -> Function-Call Split4/1
  Function-Call Split/2 -> Function-Call Split1/1

== system c2837xD_lcd_display/Initialization/Data/LCD Data ==
  Cmd : Inport
  Function-Call Generator : simulink/Ports & Subsystems/Function-Call Generator  sample_time=-1  numberOfIterations=1  DisallowWideOutput=off
  Function-Call Split : FunctionCallSplit  NumOutputPorts=2
  Function-Call Split1 : FunctionCallSplit  NumOutputPorts=2
  SendCommand : Subsystem
  SetCmd : Subsystem  TreatAsAtomicUnit=on
  SetData : Subsystem  TreatAsAtomicUnit=on
  wires:
  Function-Call Generator/1 -> Function-Call Split/1
  Function-Call Split/1 -> SetCmd/Trigger
  Cmd/1 -> SendCommand/1(cmd)
  Function-Call Split1/1 -> SendCommand/Trigger
  Function-Call Split1/2 -> SetData/Trigger
  Function-Call Split/2 -> Function-Call Split1/1

== system c2837xD_lcd_display/Initialization/DataRegister/LCD Data ==
  Cmd : Inport
  Data : Inport  Port=2
  Function-Call Generator : simulink/Ports & Subsystems/Function-Call Generator  sample_time=-1  numberOfIterations=1  DisallowWideOutput=off
  Function-Call Split : FunctionCallSplit  NumOutputPorts=2
  Function-Call Split1 : FunctionCallSplit  NumOutputPorts=2
  Function-Call Split4 : FunctionCallSplit  NumOutputPorts=2
  SendCommand : Subsystem
  SendData : Subsystem
  SetCmd : Subsystem  TreatAsAtomicUnit=on
  SetData : Subsystem  TreatAsAtomicUnit=on
  wires:
  Function-Call Generator/1 -> Function-Call Split/1
  Function-Call Split/1 -> SetCmd/Trigger
  Cmd/1 -> SendCommand/1(cmd)
  Function-Call Split1/1 -> SendCommand/Trigger
  Data/1 -> SendData/1(Data)
  Function-Call Split4/2 -> SendData/Trigger
  Function-Call Split4/1 -> SetData/Trigger
  Function-Call Split1/2 -> Function-Call Split4/1
  Function-Call Split/2 -> Function-Call Split1/1

== system c2837xD_lcd_display/Initialization/Delay1ms/System Outputs ==

== system c2837xD_lcd_display/Initialization/Delay1ms1/System Outputs ==

== system c2837xD_lcd_display/Initialization/Delay30ms/System Outputs ==

== system c2837xD_lcd_display/Initialization/DisableSPIDMA/Disable SPIDMAA ==

== system c2837xD_lcd_display/Initialization/DispEnable/Subsystem ==
  Cmd : Inport
  Data : Inport  Port=2
  Function-Call Generator : simulink/Ports & Subsystems/Function-Call Generator  sample_time=-1  numberOfIterations=1  DisallowWideOutput=off
  Function-Call Split : FunctionCallSplit  NumOutputPorts=2
  Function-Call Split1 : FunctionCallSplit  NumOutputPorts=2
  Function-Call Split4 : FunctionCallSplit  NumOutputPorts=2
  SendCommand : Subsystem
  SendData : Subsystem
  SetCmd : Subsystem  TreatAsAtomicUnit=on
  SetData : Subsystem  TreatAsAtomicUnit=on
  wires:
  Function-Call Split1/1 -> SendCommand/Trigger
  Function-Call Generator/1 -> Function-Call Split/1
  Function-Call Split/1 -> SetCmd/Trigger
  Function-Call Split4/2 -> SendData/Trigger
  Function-Call Split4/1 -> SetData/Trigger
  Data/1 -> SendData/1(Data)
  Cmd/1 -> SendCommand/1(cmd)
  Function-Call Split1/2 -> Function-Call Split4/1
  Function-Call Split/2 -> Function-Call Split1/1

== system c2837xD_lcd_display/Initialization/DispOrient/Subsystem ==
  Cmd : Inport
  Data : Inport  Port=2
  Function-Call Generator : simulink/Ports & Subsystems/Function-Call Generator  sample_time=-1  numberOfIterations=1  DisallowWideOutput=off
  Function-Call Split : FunctionCallSplit  NumOutputPorts=2
  Function-Call Split1 : FunctionCallSplit  NumOutputPorts=2
  Function-Call Split4 : FunctionCallSplit  NumOutputPorts=2
  SendCommand : Subsystem
  SendData : Subsystem
  SetCmd : Subsystem  TreatAsAtomicUnit=on
  SetData : Subsystem  TreatAsAtomicUnit=on
  wires:
  Function-Call Split1/1 -> SendCommand/Trigger
  Function-Call Generator/1 -> Function-Call Split/1
  Function-Call Split/1 -> SetCmd/Trigger
  Function-Call Split4/2 -> SendData/Trigger
  Function-Call Split4/1 -> SetData/Trigger
  Data/1 -> SendData/1(Data)
  Cmd/1 -> SendCommand/1(cmd)
  Function-Call Split1/2 -> Function-Call Split4/1
  Function-Call Split/2 -> Function-Call Split1/1

== system c2837xD_lcd_display/Initialization/EnableSCIInterrupt/SPISettings ==

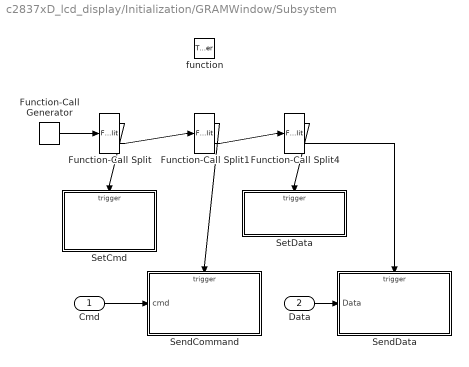
== system c2837xD_lcd_display/Initialization/GRAMWindow/Subsystem ==
  Cmd : Inport
  Data : Inport  Port=2
  function : TriggerPort  TriggerType=function-call  VariantControl=Variant
  Function-Call Generator : simulink/Ports & Subsystems/Function-Call Generator  sample_time=-1  numberOfIterations=1  DisallowWideOutput=off
  Function-Call Split : FunctionCallSplit  NumOutputPorts=2
  Function-Call Split1 : FunctionCallSplit  NumOutputPorts=2
  Function-Call Split4 : FunctionCallSplit  NumOutputPorts=2
  SendCommand : Subsystem
  SendData : Subsystem
  SetCmd : Subsystem  TreatAsAtomicUnit=on
  SetData : Subsystem  TreatAsAtomicUnit=on
  wires:
  Function-Call Split1/2 -> Function-Call Split4/1
  Function-Call Split/2 -> Function-Call Split1/1
  Data/1 -> SendData/1(Data)
  Function-Call Generator/1 -> Function-Call Split/1
  Function-Call Split/1 -> SetCmd/Trigger
  Function-Call Split4/2 -> SendData/Trigger
  Function-Call Split4/1 -> SetData/Trigger
  Function-Call Split1/1 -> SendCommand/Trigger
  Cmd/1 -> SendCommand/1(cmd)

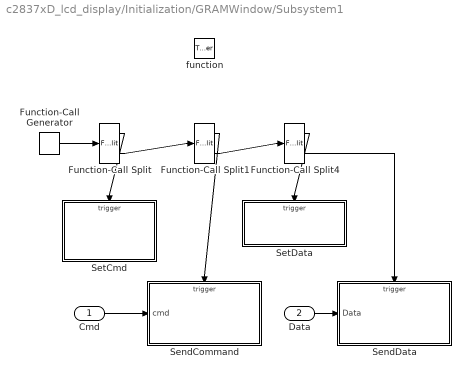
== system c2837xD_lcd_display/Initialization/GRAMWindow/Subsystem1 ==
  Cmd : Inport
  Data : Inport  Port=2
  function : TriggerPort  TriggerType=function-call  VariantControl=Variant
  Function-Call Generator : simulink/Ports & Subsystems/Function-Call Generator  sample_time=-1  numberOfIterations=1  DisallowWideOutput=off
  Function-Call Split : FunctionCallSplit  NumOutputPorts=2
  Function-Call Split1 : FunctionCallSplit  NumOutputPorts=2
  Function-Call Split4 : FunctionCallSplit  NumOutputPorts=2
  SendCommand : Subsystem
  SendData : Subsystem
  SetCmd : Subsystem  TreatAsAtomicUnit=on
  SetData : Subsystem  TreatAsAtomicUnit=on
  wires:
  Function-Call Split1/2 -> Function-Call Split4/1
  Function-Call Split/2 -> Function-Call Split1/1
  Data/1 -> SendData/1(Data)
  Function-Call Generator/1 -> Function-Call Split/1
  Function-Call Split/1 -> SetCmd/Trigger
  Function-Call Split4/2 -> SendData/Trigger
  Function-Call Split4/1 -> SetData/Trigger
  Function-Call Split1/1 -> SendCommand/Trigger
  Cmd/1 -> SendCommand/1(cmd)

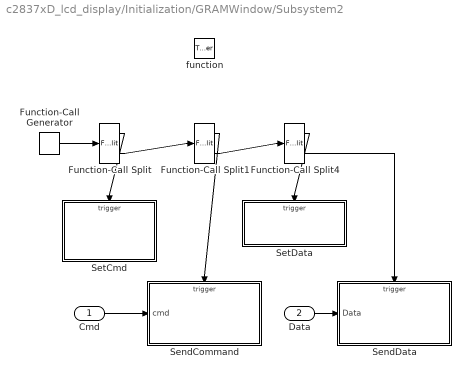
== system c2837xD_lcd_display/Initialization/GRAMWindow/Subsystem2 ==
  Cmd : Inport
  Data : Inport  Port=2
  function : TriggerPort  TriggerType=function-call  VariantControl=Variant
  Function-Call Generator : simulink/Ports & Subsystems/Function-Call Generator  sample_time=-1  numberOfIterations=1  DisallowWideOutput=off
  Function-Call Split : FunctionCallSplit  NumOutputPorts=2
  Function-Call Split1 : FunctionCallSplit  NumOutputPorts=2
  Function-Call Split4 : FunctionCallSplit  NumOutputPorts=2
  SendCommand : Subsystem
  SendData : Subsystem
  SetCmd : Subsystem  TreatAsAtomicUnit=on
  SetData : Subsystem  TreatAsAtomicUnit=on
  wires:
  Function-Call Split1/2 -> Function-Call Split4/1
  Function-Call Split/2 -> Function-Call Split1/1
  Data/1 -> SendData/1(Data)
  Function-Call Generator/1 -> Function-Call Split/1
  Function-Call Split/1 -> SetCmd/Trigger
  Function-Call Split4/2 -> SendData/Trigger
  Function-Call Split4/1 -> SetData/Trigger
  Function-Call Split1/1 -> SendCommand/Trigger
  Cmd/1 -> SendCommand/1(cmd)

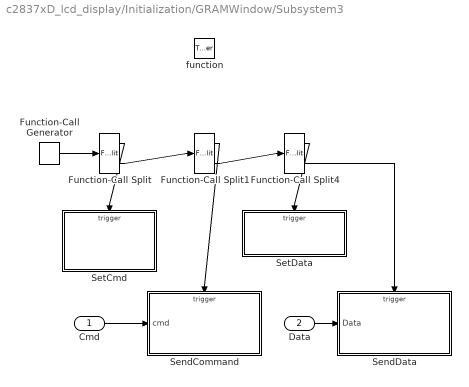
== system c2837xD_lcd_display/Initialization/GRAMWindow/Subsystem3 ==
  Cmd : Inport
  Data : Inport  Port=2
  function : TriggerPort  TriggerType=function-call  VariantControl=Variant
  Function-Call Generator : simulink/Ports & Subsystems/Function-Call Generator  sample_time=-1  numberOfIterations=1  DisallowWideOutput=off
  Function-Call Split : FunctionCallSplit  NumOutputPorts=2
  Function-Call Split1 : FunctionCallSplit  NumOutputPorts=2
  Function-Call Split4 : FunctionCallSplit  NumOutputPorts=2
  SendCommand : Subsystem
  SendData : Subsystem
  SetCmd : Subsystem  TreatAsAtomicUnit=on
  SetData : Subsystem  TreatAsAtomicUnit=on
  wires:
  Function-Call Split1/2 -> Function-Call Split4/1
  Function-Call Split/2 -> Function-Call Split1/1
  Data/1 -> SendData/1(Data)
  Function-Call Generator/1 -> Function-Call Split/1
  Function-Call Split/1 -> SetCmd/Trigger
  Function-Call Split4/2 -> SendData/Trigger
  Function-Call Split4/1 -> SetData/Trigger
  Function-Call Split1/1 -> SendCommand/Trigger
  Cmd/1 -> SendCommand/1(cmd)

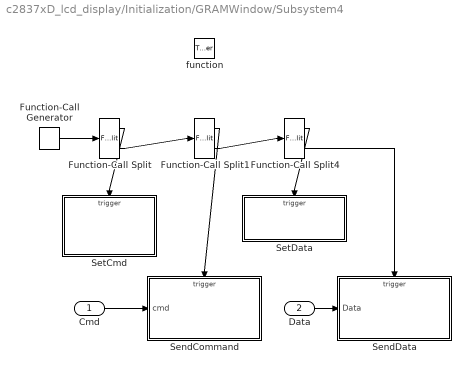
== system c2837xD_lcd_display/Initialization/GRAMWindow/Subsystem4 ==
  Cmd : Inport
  Data : Inport  Port=2
  function : TriggerPort  TriggerType=function-call  VariantControl=Variant
  Function-Call Generator : simulink/Ports & Subsystems/Function-Call Generator  sample_time=-1  numberOfIterations=1  DisallowWideOutput=off
  Function-Call Split : FunctionCallSplit  NumOutputPorts=2
  Function-Call Split1 : FunctionCallSplit  NumOutputPorts=2
  Function-Call Split4 : FunctionCallSplit  NumOutputPorts=2
  SendCommand : Subsystem
  SendData : Subsystem
  SetCmd : Subsystem  TreatAsAtomicUnit=on
  SetData : Subsystem  TreatAsAtomicUnit=on
  wires:
  Function-Call Split1/2 -> Function-Call Split4/1
  Function-Call Split/2 -> Function-Call Split1/1
  Data/1 -> SendData/1(Data)
  Function-Call Generator/1 -> Function-Call Split/1
  Function-Call Split/1 -> SetCmd/Trigger
  Function-Call Split4/2 -> SendData/Trigger
  Function-Call Split4/1 -> SetData/Trigger
  Function-Call Split1/1 -> SendCommand/Trigger
  Cmd/1 -> SendCommand/1(cmd)

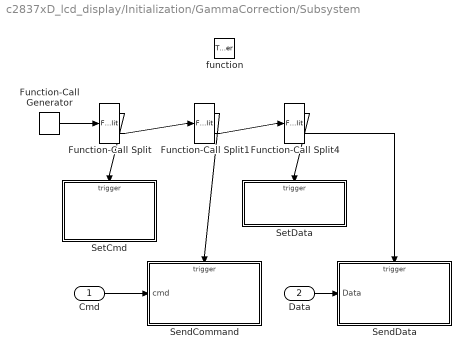
== system c2837xD_lcd_display/Initialization/GammaCorrection/Subsystem ==
  Cmd : Inport
  Data : Inport  Port=2
  function : TriggerPort  TriggerType=function-call  VariantControl=Variant
  Function-Call Generator : simulink/Ports & Subsystems/Function-Call Generator  sample_time=-1  numberOfIterations=1  DisallowWideOutput=off
  Function-Call Split : FunctionCallSplit  NumOutputPorts=2
  Function-Call Split1 : FunctionCallSplit  NumOutputPorts=2
  Function-Call Split4 : FunctionCallSplit  NumOutputPorts=2
  SendCommand : Subsystem
  SendData : Subsystem
  SetCmd : Subsystem  TreatAsAtomicUnit=on
  SetData : Subsystem  TreatAsAtomicUnit=on
  wires:
  Function-Call Split1/2 -> Function-Call Split4/1
  Function-Call Split/2 -> Function-Call Split1/1
  Data/1 -> SendData/1(Data)
  Function-Call Generator/1 -> Function-Call Split/1
  Function-Call Split/1 -> SetCmd/Trigger
  Function-Call Split4/2 -> SendData/Trigger
  Function-Call Split4/1 -> SetData/Trigger
  Function-Call Split1/1 -> SendCommand/Trigger
  Cmd/1 -> SendCommand/1(cmd)

== system c2837xD_lcd_display/Initialization/GammaCorrection/Subsystem1 ==
  Cmd : Inport
  Data : Inport  Port=2
  function : TriggerPort  TriggerType=function-call  VariantControl=Variant
  Function-Call Generator : simulink/Ports & Subsystems/Function-Call Generator  sample_time=-1  numberOfIterations=1  DisallowWideOutput=off
  Function-Call Split : FunctionCallSplit  NumOutputPorts=2
  Function-Call Split1 : FunctionCallSplit  NumOutputPorts=2
  Function-Call Split4 : FunctionCallSplit  NumOutputPorts=2
  SendCommand : Subsystem
  SendData : Subsystem
  SetCmd : Subsystem  TreatAsAtomicUnit=on
  SetData : Subsystem  TreatAsAtomicUnit=on
  wires:
  Function-Call Split1/2 -> Function-Call Split4/1
  Function-Call Split/2 -> Function-Call Split1/1
  Data/1 -> SendData/1(Data)
  Function-Call Generator/1 -> Function-Call Split/1
  Function-Call Split/1 -> SetCmd/Trigger
  Function-Call Split4/2 -> SendData/Trigger
  Function-Call Split4/1 -> SetData/Trigger
  Function-Call Split1/1 -> SendCommand/Trigger
  Cmd/1 -> SendCommand/1(cmd)

== system c2837xD_lcd_display/Initialization/GammaCorrection/Subsystem2 ==
  Cmd : Inport
  Data : Inport  Port=2
  function : TriggerPort  TriggerType=function-call  VariantControl=Variant
  Function-Call Generator : simulink/Ports & Subsystems/Function-Call Generator  sample_time=-1  numberOfIterations=1  DisallowWideOutput=off
  Function-Call Split : FunctionCallSplit  NumOutputPorts=2
  Function-Call Split1 : FunctionCallSplit  NumOutputPorts=2
  Function-Call Split4 : FunctionCallSplit  NumOutputPorts=2
  SendCommand : Subsystem
  SendData : Subsystem
  SetCmd : Subsystem  TreatAsAtomicUnit=on
  SetData : Subsystem  TreatAsAtomicUnit=on
  wires:
  Function-Call Split1/2 -> Function-Call Split4/1
  Function-Call Split/2 -> Function-Call Split1/1
  Data/1 -> SendData/1(Data)
  Function-Call Generator/1 -> Function-Call Split/1
  Function-Call Split/1 -> SetCmd/Trigger
  Function-Call Split4/2 -> SendData/Trigger
  Function-Call Split4/1 -> SetData/Trigger
  Function-Call Split1/1 -> SendCommand/Trigger
  Cmd/1 -> SendCommand/1(cmd)

== system c2837xD_lcd_display/Initialization/GammaCorrection/Subsystem3 ==
  Cmd : Inport
  Data : Inport  Port=2
  function : TriggerPort  TriggerType=function-call  VariantControl=Variant
  Function-Call Generator : simulink/Ports & Subsystems/Function-Call Generator  sample_time=-1  numberOfIterations=1  DisallowWideOutput=off
  Function-Call Split : FunctionCallSplit  NumOutputPorts=2
  Function-Call Split1 : FunctionCallSplit  NumOutputPorts=2
  Function-Call Split4 : FunctionCallSplit  NumOutputPorts=2
  SendCommand : Subsystem
  SendData : Subsystem
  SetCmd : Subsystem  TreatAsAtomicUnit=on
  SetData : Subsystem  TreatAsAtomicUnit=on
  wires:
  Function-Call Split1/2 -> Function-Call Split4/1
  Function-Call Split/2 -> Function-Call Split1/1
  Data/1 -> SendData/1(Data)
  Function-Call Generator/1 -> Function-Call Split/1
  Function-Call Split/1 -> SetCmd/Trigger
  Function-Call Split4/2 -> SendData/Trigger
  Function-Call Split4/1 -> SetData/Trigger
  Function-Call Split1/1 -> SendCommand/Trigger
  Cmd/1 -> SendCommand/1(cmd)

== system c2837xD_lcd_display/Initialization/GammaCorrection/Subsystem4 ==
  Cmd : Inport
  Data : Inport  Port=2
  function : TriggerPort  TriggerType=function-call  VariantControl=Variant
  Function-Call Generator : simulink/Ports & Subsystems/Function-Call Generator  sample_time=-1  numberOfIterations=1  DisallowWideOutput=off
  Function-Call Split : FunctionCallSplit  NumOutputPorts=2
  Function-Call Split1 : FunctionCallSplit  NumOutputPorts=2
  Function-Call Split4 : FunctionCallSplit  NumOutputPorts=2
  SendCommand : Subsystem
  SendData : Subsystem
  SetCmd : Subsystem  TreatAsAtomicUnit=on
  SetData : Subsystem  TreatAsAtomicUnit=on
  wires:
  Function-Call Split1/2 -> Function-Call Split4/1
  Function-Call Split/2 -> Function-Call Split1/1
  Data/1 -> SendData/1(Data)
  Function-Call Generator/1 -> Function-Call Split/1
  Function-Call Split/1 -> SetCmd/Trigger
  Function-Call Split4/2 -> SendData/Trigger
  Function-Call Split4/1 -> SetData/Trigger
  Function-Call Split1/1 -> SendCommand/Trigger
  Cmd/1 -> SendCommand/1(cmd)

== system c2837xD_lcd_display/Initialization/GammaCorrection1/Subsystem ==
  Cmd : Inport
  Data : Inport  Port=2
  function : TriggerPort  TriggerType=function-call  VariantControl=Variant
  Function-Call Generator : simulink/Ports & Subsystems/Function-Call Generator  sample_time=-1  numberOfIterations=1  DisallowWideOutput=off
  Function-Call Split : FunctionCallSplit  NumOutputPorts=2
  Function-Call Split1 : FunctionCallSplit  NumOutputPorts=2
  Function-Call Split4 : FunctionCallSplit  NumOutputPorts=2
  SendCommand : Subsystem
  SendData : Subsystem
  SetCmd : Subsystem  TreatAsAtomicUnit=on
  SetData : Subsystem  TreatAsAtomicUnit=on
  wires:
  Function-Call Split1/2 -> Function-Call Split4/1
  Function-Call Split/2 -> Function-Call Split1/1
  Data/1 -> SendData/1(Data)
  Function-Call Generator/1 -> Function-Call Split/1
  Function-Call Split/1 -> SetCmd/Trigger
  Function-Call Split4/2 -> SendData/Trigger
  Function-Call Split4/1 -> SetData/Trigger
  Function-Call Split1/1 -> SendCommand/Trigger
  Cmd/1 -> SendCommand/1(cmd)
